simulink model "pdmRecipPump"  (R2021b)
settings: Solver=VariableStepAuto  StartTime=0.0  StopTime=2  RelTol=1e-3  EnableMultiTasking=on
undefined symbols (not defined in the file or in its folder): bearing_fault_frict_WKSP, bearing_visc_frict_WKSP, block_in_factor_WKSP, chkv_in_maxA_WKSP, noise_seed_offset_WKSP, smiData, TRP_Par, X, Y, Z
libraries: sm_lib x71, fl_lib x30, nesl_utility x13, sh_lib x8, simulink x7, ee_lib x2, Mech_Hydro_Elec_Multibody_Lib x2, sm_pump_triplex_lib x2
(part 2 of 4)

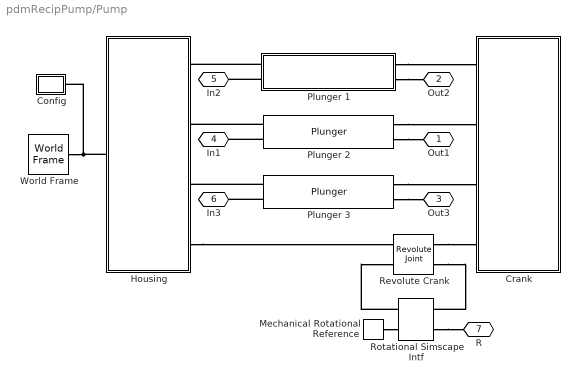
== system pdmRecipPump/Pump ==
  Config : Subsystem
  Crank : Subsystem  mask(Crankshaft){shaft_len=shaft_len_P, shaft_rad=shaft_rad_P, web_rad=web_rad_P, web_len=web_len_P, motor_shaft_rad=motor_shaft_rad_P, motor_shaft_len=motor_shaft_len_P, shaft_pos=shaft_pos_P, crank_rho=crank_rho_P, motor_shaft_clr=motor_shaft_clr_P, crank_clr=crank_clr_P, crank_opc=crank_opc_P}
      mask prompts: shaft_pos "Crankpin Axis Offset (m)"; crank_rho "Density (kg/m^3)"; motor_shaft_clr "Motor Shaft Color [RGB]"; crank_clr "Crank Color [RGB]"; crank_opc "Opacity (0-1)"
      mask help: Models pump crankshaft with three crankpins, each offset by 120 degrees from the crankshaft axis.
      mask DialogControl text_radius Prompt: Radius (m)
      mask DialogControl text_length Prompt: Length (m)
      mask DialogControl text_crankpin Prompt: Crankpin
      mask DialogControl text_web Prompt: Web
      mask DialogControl text_motor_shaft Prompt: Motor Shaft
      mask DialogControl cont_crank_vis Prompt: Crankshaft Visualization
      mask Display: image('sm_pump_triplex_Crank_IMAGE.png');
  Housing : Subsystem
      mask Display: image('sm_pump_triplex_Housing_IMAGE.png');
  Mechanical Rotational Reference : fl_lib/Mechanical/Rotational Elements/Mechanical Rotational Reference
  Plunger 1 : Subsystem  mask(Hydraulic Plunger){cyl_gap=cyl_gap_P, cyl_rad_out=cyl_rad_out_P, cyl_len=cyl_len_P, cyl_stroke=cyl_stroke_P, cyl_rad_in=0, cyl_xc_rev=0, cyl_frict_brkway_frc=cyl_frict_brkway_frc_P, cyl_frict_brkway_vel=cyl_frict_brkway_vel_P, cyl_frict_col_frc=cyl_frict_col_frc_P, cyl_frict_visc_coef=cyl_frict_visc_coef_P, cyl_rho=cyl_rho_P, cyl_clr=cyl_clr_P, cyl_opc=cyl_opc_P, cyl_xc=0, plgB_len=plgB_len_P, plgB_rad=plgB_rad_P, stem_len=stem_len_P, stem_rad=stem_rad_P, pin_len=pin_len_P, pin_rad=pin_rad_P, cup_rad_out=cup_rad_out_P, cup_thk=cup_thk_P, cup_len=cup_len_P, cup_pinOffset=cup_pinOffset_P, cup_rad_in=0, plg_rho=plg_rho_P, plg_clr=plg_clr_P, plg_opc=plg_opc_P, conrod_len=conrod_len_P, conrod_web_widP=conrod_web_widP_P, conrod_web_widC=conrod_web_widC_P, conrod_web_offC=0, conrod_web_offP=0, conrod_web_len=0, conrod_web_xc=0, conrod_ringC_wid=conrod_ringC_wid_P, conrod_ringP_wid=conrod_ringP_wid_P, crank_shaft_rad=crank_shaft_rad_P, conrod_ringC_or=0, conrod_ringP_or=0, conrod_ringC_xc_rev=0, conrod_ringP_xc_rev=0, conrod_thk=conrod_thk_P, conrod_rho=conrod_rho_P, conrod_clr=conrod_clr_P, conrod_opc=conrod_opc_P, chkv_in_maxA=chkv_in_maxA_P, chkv_out_maxA=chkv_out_maxA_P, chkv_in_crkP=chkv_in_crkP_P, chkv_out_crkP=chkv_out_crkP_P, chkv_in_maxOpenP=chkv_in_maxOpenP_P, chkv_out_maxOpenP=chkv_out_maxOpenP_P, chkv_vis_popup=Off, chkv_vis_rad_in=chkv_vis_rad_in_P, chkv_vis_rad_out=chkv_vis_rad_out_P, chkv_vis_clr_in=chkv_vis_clr_in_P, chkv_vis_clr_out=chkv_vis_clr_out_P, leak_cyl_popup=On, Run Time, leak_cyl_area=leak_cyl1_area, block_in_popup=On, Run Time, block_in_factor=block_in_cyl1_factor, seal_leak_vis_len=seal_leak_vis_len_P, seal_leak_vis_rad=seal_leak_vis_rad_P, seal_leak_vis_clr=seal_leak_vis_clr_P, seal_leak_vis_opc=0, inlet_obstr_len=inlet_obstr_len_P, inlet_obstr_rad=inlet_obstr_rad_P, inlet_obstr_xc_rev=0, inlet_obstr_clr=inlet_obstr_clr_P, inlet_obstr_opc=1}
      mask prompts: cyl_gap "Gap (m)"; cyl_rad_out "Outer radius (m)"; cyl_len "Length (m)"; cyl_stroke "Stroke (m)"; cyl_rad_in "Inner radius (m)"; cyl_xc_rev "Revolution Cross Section (m)"; cyl_frict_brkway_frc "Breakaway Friction Force (N)"; cyl_frict_brkway_vel "Breakaway Friction Velocity (m/s)"; cyl_frict_col_frc "Coulomb Friction Force (N)"; cyl_frict_visc_coef "Viscous Friction Coeff (N/(m/s))"; cyl_rho "Density (kg/m^3)"; cyl_clr "Color [RGB]"; cyl_opc "Opacity (0-1)"; cyl_xc "Cylinder Cross Section (m)"; cup_rad_out "Outer Radius (m)"; cup_thk "Wall Thickness (m)"; cup_len "Length(m)"; cup_pinOffset "Pin Offset (m)"; cup_rad_in "Inner Radius (m)"; plg_rho "Density (kg/m^3)"; plg_clr "Color [RGB]"; plg_opc "Opacity (0-1)"; conrod_len "Length, center-center (m)"; conrod_web_widP "Width, pin end (m)"; conrod_web_widC "Width, crank end (m)"; conrod_web_offC "Offset to shaft center (m)"; conrod_web_offP "Offset to pin center (m)"; conrod_web_len "Length web (m)"; conrod_web_xc "Extrusion cross section (m)"; conrod_ringC_wid "Crank Ring Width (m)"; conrod_ringP_wid "Pin Ring Width (m)"; crank_shaft_rad "Crank Shaft Radius (m)"; conrod_ringC_or "Outer Radius, Crank Ring"; conrod_ringP_or "Inner Radius, Pin Ring"; conrod_ringC_xc_rev "Crank Ring Cross Section (m)"; conrod_ringP_xc_rev "Pin Ring Cross Section (m)"; conrod_thk "Thickness (m)"; conrod_rho "Density (kg/m^3)"; conrod_clr "Color [RGB]"; conrod_opc "Opacity (0-1)"; chkv_vis_popup "Valve Visualization"; leak_cyl_popup "Seal Leak"; leak_cyl_area "Leak Area (m^2)"; block_in_popup "Blocked Inlet"; block_in_factor "Area Factor (0-1)"; seal_leak_vis_len "Length (m)"; seal_leak_vis_rad "Radius (m)"; seal_leak_vis_clr "Color [RGB]"; seal_leak_vis_opc "Opacity (0-1)"; inlet_obstr_len "Length (m)"; inlet_obstr_rad "Radius (m)"; inlet_obstr_xc_rev "Cross Section (m)"; inlet_obstr_clr "Color [RGB]"; inlet_obstr_opc "Opacity (0-1)"
      mask help: Models a single hydraulic plunger with hydraulic chamber. Two check valves control flow into and out of the hydraulic chamber. Degraded behavior can be modeled by enabling seal leakage and blocked inlet on the Faults tab. When "On, Run Time" is selected, MATLAB workspace variables set the parameters so that they can be tuned using Fast Restart.
      mask init:
      | % -- Configure submodels
      | % Fault: Seal Leak
      | if(leak_cyl_popup==1)
      |     set_param([gcb '/Seal Leak'],'OverrideUsingVariant','Off');
      |     seal_leak_vis_opc = 0;
      | elseif(leak_cyl_popup==2)
      |     set_param([gcb '/Seal Leak'],'OverrideUsingVariant','On');
      |     seal_leak_vis_opc = 1;
      | elseif(leak_cyl_popup==3)
      |     set_param([gcb '/Seal Leak'],'OverrideUsingVariant','Tune');
      |     seal_leak_vis_opc = 1;
      | end
      | 
      | % Fault: Blocked Inlet
      | inlet_obstr_xc_rev = [...
      |     inlet_obstr_rad                  -inlet_obstr_len/2;
      |     inlet_obstr_rad                   inlet_obstr_len/2;
      |     inlet_obstr_rad*block_in_factor   inlet_obstr_len/2;
      |     inlet_obstr_rad*block_in_factor  -inlet_obstr_len/2];
      | if(block_in_popup==1)
      |     set_param([gcb '/Check Valve Inlet'],...
      |         'area_max','chkv_in_maxA',...
      |         'area_max_conf','compiletime',...
      |         'BackgroundColor','[1 1 1]');
      |     inlet_obstr_opc = 0;
      | elseif(block_in_popup==2)
      |     set_param([gcb '/Check Valve Inlet'],...
      |         'area_max','chkv_in_maxA*block_in_factor',...
      |         'area_max_conf','compiletime',...
      |         'BackgroundColor','[1 0.9 0.9]');
      |     inlet_obstr_opc = 1;
      | elseif(block_in_popup==3)
      |     set_param([gcb '/Check Valve Inlet'],...
      |         'area_max','chkv_in_maxA_WKSP*block_in_factor_WKSP',...
      |         'area_max_conf','runtime',...
      |         'BackgroundColor','[1 0.9 0.9]');
      |     inlet_obstr_opc = 1;
      | end
      | 
      | % Turn on/off visualization
      | if(chkv_vis_popup==1)
      |     set_param([gcb '/Valve Visual'],'OverrideUsingVariant','Off');
      | elseif(chkv_vis_popup==2)
      |     set_param([gcb '/Valve Visual'],'OverrideUsingVariant','On');
      | end    
      | 
      | % -- Calculate derived parameters
      | % Cylinder: derived dimensions
      | cyl_rad_in  = plgB_rad + cyl_gap;
      | %cyl_len     = crank_shaft_pos*2+plgB_len;
      | 
      | % Cylinder: cross-section for rev
      | cyl_xc_rev = [...
      |     cyl_rad_out  -cyl_len/2
      |     cyl_rad_out   cyl_len/2
      |     cyl_rad_in    cyl_len/2
      |     cyl_rad_in   -cyl_len/2];
      | 
      | % Stem Cup: cross-section for rev
      | cup_rad_in = cup_rad_out-cup_thk;
      | cup_xc_rev = [...
      |     cup_rad_out  -cup_len/2
      |     cup_rad_out   cup_len/2
      |     cup_rad_in    cup_len/2
      |     cup_rad_in   -cup_len/2];
      | 
      | % Connecting Rod, Crank Ring: cross-section for rev
      | conrod_ringC_or = crank_shaft_rad + conrod_ringC_wid;
      | conrod_ringC_xc_rev = [...
      |     conrod_ringC_or -conrod_thk/2*1.005;
      |     conrod_ringC_or  conrod_thk/2*1.005;
      |     crank_shaft_rad  conrod_thk/2*1.005;
      |     crank_shaft_rad -conrod_thk/2*1.005];
      | 
      | % Connecting Rod, Pin ring: cross-section for rev
      | conrod_ringP_or = pin_rad + conrod_ringP_wid;
      | conrod_ringP_xc_rev = [...
      |     conrod_ringP_or -conrod_thk/2*1.005;
      |     conrod_ringP_or  conrod_thk/2*1.005;
      |     pin_rad          conrod_thk/2*1.005;
      |     pin_rad         -conrod_thk/2*1.005];
      | 
      | % Connecting Rod, Web: cross-section for extrusion
      | conrod_web_offC = crank_shaft_rad + conrod_ringC_wid/2;
      | conrod_web_offP = pin_rad         + conrod_ringP_wid/2;
      | conrod_web_len  = conrod_len - conrod_web_offP - conrod_web_offC;
      | conrod_web_xc = [...
      |     -conrod_web_len -conrod_web_widC;
      |      conrod_web_len -conrod_web_widP;
      |      conrod_web_len  conrod_web_widP;
      |     -conrod_web_len  conrod_web_widC]/2;
      mask TypeOptions chkv_vis_popup: Off | On
      mask TypeOptions leak_cyl_popup: Off | On | On, Run Time
      mask Callback leak_cyl_popup:
      | maskObj = Simulink.Mask.get(gcb);
      | leak_area_h = maskObj.getParameter('leak_cyl_area');
      | leak_text_h = maskObj.getDialogControl('leak_cyl_tune_text');
      | if (strcmp(get_param(gcb,'leak_cyl_popup'),'Off'))
      |     leak_area_h.Visible = 'off';
      |     leak_text_h.Visible = 'off';
      | elseif (strcmp(get_param(gcb,'leak_cyl_popup'),'On'))
      |     leak_area_h.Visible = 'on';
      |     leak_text_h.Visible = 'off';
      | elseif (strcmp(get_param(gcb,'leak_cyl_popup'),'On, Run Time'))
      |     leak_area_h.Visible = 'off';
      |     leak_text_h.Visible = 'on';
      | end
      | %clear maskObj leak_area_h leak_text_h
      mask TypeOptions block_in_popup: Off | On | On, Run Time
      mask Callback block_in_popup:
      | maskObj = Simulink.Mask.get(gcb);
      | block_fctr_h = maskObj.getParameter('block_in_factor');
      | block_text_h = maskObj.getDialogControl('block_in_tune_text');
      | if (strcmp(get_param(gcb,'block_in_popup'),'Off'))
      |     block_fctr_h.Visible = 'off';
      |     block_text_h.Visible = 'off';
      | elseif (strcmp(get_param(gcb,'block_in_popup'),'On'))
      |     block_fctr_h.Visible = 'on';
      |     block_text_h.Visible = 'off';
      | elseif (strcmp(get_param(gcb,'block_in_popup'),'On, Run Time'))
      |     block_fctr_h.Visible = 'off';
      |     block_text_h.Visible = 'on';
      | end
      | clear maskObj block_fctr_h block_text_h
      mask DialogControl tab_cylinder Prompt: Cylinder
      mask DialogControl cont_dims Prompt: Dimensions
      mask DialogControl cont_friction Prompt: Friction
      mask DialogControl tab_plunger Prompt: Plunger
      mask DialogControl text_length Prompt: Length (m)
      mask DialogControl text_radius Prompt: Radius (m)
      mask DialogControl text_base Prompt: Base
      mask DialogControl text_stem Prompt: Stem
      mask DialogControl text_pin Prompt: Pin
      mask DialogControl cont_cup Prompt: Cup
      mask DialogControl cont_plg_vis Prompt: Plunger Visualization
      mask DialogControl tab_conrod Prompt: Rod
      mask DialogControl cont_conrodWeb Prompt: Web
      mask DialogControl cont_conrodRings Prompt: Rings
      mask DialogControl cont_conrod_vis Prompt: Rod Visualization
      mask DialogControl tab_valves Prompt: Valves
      mask DialogControl text_open_inlet Prompt: Inlet
      mask DialogControl text_open_outlet Prompt: Outlet
      mask DialogControl text_open_maxA Prompt: Max Area (m)
      mask DialogControl text_open_crkP Prompt: Crack. Pr (Pa)
      mask DialogControl text_open_maxOpenP Prompt: Max Open. Pr. (Pa)
      mask DialogControl cont_valve_vis Prompt: Visualization Settings
      mask DialogControl text_valvis_inlet Prompt: Inlet
      mask DialogControl text_valvis_out Prompt: Outlet
      mask DialogControl text_valvis_rad Prompt: Radius (m)
      mask DialogControl text_valvis_clr Prompt: Color [RGB]
      mask DialogControl tab_faults Prompt: Faults
      mask DialogControl leak_cyl_tune_text Prompt: Set >> leak_cyl_area_WKSP
      mask DialogControl block_in_tune_text Prompt: Set >> block_in_factor_WKSP, chkv_out_maxA_WKSP
      mask DialogControl cont_seal_leak_vis Prompt: Seal Leak Visualization
      mask DialogControl cont_blocked_line_vis Prompt: Blocked Line Visualization
      mask Display: image('sm_pump_triplex_Plunger_IMAGE.png');
  Plunger 2 : sm_pump_triplex_lib/Plunger  cyl_gap=cyl_gap_P  cyl_rad_out=cyl_rad_out_P  cyl_len=cyl_len_P  cyl_stroke=cyl_stroke_P  cyl_rad_in=0  cyl_xc_rev=0  cyl_frict_brkway_frc=cyl_frict_brkway_frc_P  cyl_frict_brkway_vel=cyl_frict_brkway_vel_P  cyl_frict_col_frc=cyl_frict_col_frc_P  cyl_frict_visc_coef=cyl_frict_visc_coef_P  cyl_rho=cyl_rho_P  cyl_clr=cyl_clr_P  cyl_opc=cyl_opc_P  cyl_xc=0  plgB_len=plgB_len_P  plgB_rad=plgB_rad_P  stem_len=stem_len_P  stem_rad=stem_rad_P  pin_len=pin_len_P  pin_rad=pin_rad_P  cup_rad_out=cup_rad_out_P  cup_thk=cup_thk_P  cup_len=cup_len_P  cup_pinOffset=cup_pinOffset_P  cup_rad_in=0  plg_rho=plg_rho_P  plg_clr=plg_clr_P  plg_opc=plg_opc_P  conrod_len=conrod_len_P  conrod_web_widP=conrod_web_widP_P  conrod_web_widC=conrod_web_widC_P  conrod_web_offC=0  conrod_web_offP=0  conrod_web_len=0  conrod_web_xc=0  conrod_ringC_wid=conrod_ringC_wid_P  conrod_ringP_wid=conrod_ringP_wid_P  crank_shaft_rad=crank_shaft_rad_P  conrod_ringC_or=0  conrod_ringP_or=0  conrod_ringC_xc_rev=0  conrod_ringP_xc_rev=0  conrod_thk=conrod_thk_P  conrod_rho=conrod_rho_P  conrod_clr=conrod_clr_P  conrod_opc=conrod_opc_P  chkv_in_maxA=chkv_in_maxA_P  chkv_out_maxA=chkv_out_maxA_P  chkv_in_crkP=chkv_in_crkP_P  chkv_out_crkP=chkv_out_crkP_P  chkv_in_maxOpenP=chkv_in_maxOpenP_P  chkv_out_maxOpenP=chkv_out_maxOpenP_P  chkv_vis_popup=Off  chkv_vis_rad_in=chkv_vis_rad_in_P  chkv_vis_rad_out=chkv_vis_rad_out_P  chkv_vis_clr_in=chkv_vis_clr_in_P  chkv_vis_clr_out=chkv_vis_clr_out_P  leak_cyl_popup=Off  leak_cyl_area=leak_cyl2_area  block_in_popup=Off  block_in_factor=block_in_cyl2_factor  seal_leak_vis_len=seal_leak_vis_len_P  seal_leak_vis_rad=seal_leak_vis_rad_P  seal_leak_vis_clr=seal_leak_vis_clr_P  seal_leak_vis_opc=0  inlet_obstr_len=inlet_obstr_len_P  inlet_obstr_rad=inlet_obstr_rad_P  inlet_obstr_xc_rev=0  inlet_obstr_clr=inlet_obstr_clr_P  inlet_obstr_opc=1
  Plunger 3 : sm_pump_triplex_lib/Plunger  cyl_gap=cyl_gap_P  cyl_rad_out=cyl_rad_out_P  cyl_len=cyl_len_P  cyl_stroke=cyl_stroke_P  cyl_rad_in=0  cyl_xc_rev=0  cyl_frict_brkway_frc=cyl_frict_brkway_frc_P  cyl_frict_brkway_vel=cyl_frict_brkway_vel_P  cyl_frict_col_frc=cyl_frict_col_frc_P  cyl_frict_visc_coef=cyl_frict_visc_coef_P  cyl_rho=cyl_rho_P  cyl_clr=cyl_clr_P  cyl_opc=cyl_opc_P  cyl_xc=0  plgB_len=plgB_len_P  plgB_rad=plgB_rad_P  stem_len=stem_len_P  stem_rad=stem_rad_P  pin_len=pin_len_P  pin_rad=pin_rad_P  cup_rad_out=cup_rad_out_P  cup_thk=cup_thk_P  cup_len=cup_len_P  cup_pinOffset=cup_pinOffset_P  cup_rad_in=0  plg_rho=plg_rho_P  plg_clr=plg_clr_P  plg_opc=plg_opc_P  conrod_len=conrod_len_P  conrod_web_widP=conrod_web_widP_P  conrod_web_widC=conrod_web_widC_P  conrod_web_offC=0  conrod_web_offP=0  conrod_web_len=0  conrod_web_xc=0  conrod_ringC_wid=conrod_ringC_wid_P  conrod_ringP_wid=conrod_ringP_wid_P  crank_shaft_rad=crank_shaft_rad_P  conrod_ringC_or=0  conrod_ringP_or=0  conrod_ringC_xc_rev=0  conrod_ringP_xc_rev=0  conrod_thk=conrod_thk_P  conrod_rho=conrod_rho_P  conrod_clr=conrod_clr_P  conrod_opc=conrod_opc_P  chkv_in_maxA=chkv_in_maxA_P  chkv_out_maxA=chkv_out_maxA_P  chkv_in_crkP=chkv_in_crkP_P  chkv_out_crkP=chkv_out_crkP_P  chkv_in_maxOpenP=chkv_in_maxOpenP_P  chkv_out_maxOpenP=chkv_out_maxOpenP_P  chkv_vis_popup=Off  chkv_vis_rad_in=chkv_vis_rad_in_P  chkv_vis_rad_out=chkv_vis_rad_out_P  chkv_vis_clr_in=chkv_vis_clr_in_P  chkv_vis_clr_out=chkv_vis_clr_out_P  leak_cyl_popup=Off  leak_cyl_area=leak_cyl3_area  block_in_popup=Off  block_in_factor=block_in_cyl3_factor  seal_leak_vis_len=seal_leak_vis_len_P  seal_leak_vis_rad=seal_leak_vis_rad_P  seal_leak_vis_clr=seal_leak_vis_clr_P  seal_leak_vis_opc=0  inlet_obstr_len=inlet_obstr_len_P  inlet_obstr_rad=inlet_obstr_rad_P  inlet_obstr_xc_rev=0  inlet_obstr_clr=inlet_obstr_clr_P  inlet_obstr_opc=1
  Revolute Crank : sm_lib/Joints/Revolute Joint  JointMode=Normal  SenseConstraintForce=off  SenseConstraintForceX=off  SenseConstraintForceY=off  SenseConstraintForceZ=off  SenseConstraintTorque=off  SenseConstraintTorqueX=off  SenseConstraintTorqueY=off  SenseConstraintTorqueZ=off  SenseTotalForce=off  SenseTotalForceX=off  SenseTotalForceY=off  SenseTotalForceZ=off  SenseTotalTorque=off  SenseTotalTorqueX=off  SenseTotalTorqueY=off  SenseTotalTorqueZ=off  CompositeWrenchDir=FollowerOnBase  CompositeWrenchFrame=BaseFrame  EquilibriumPosition=0  EquilibriumPositionUnits=deg  SpringStiffness=0  SpringStiffnessUnits=N*m/deg  DampingCoefficient=bearing_visc_frict_WKSP+bearing_fault_frict_WKSP  DampingCoefficientUnits=N*m/(deg/s)  TorqueActuationMode=InputTorque  MotionActuationMode=ComputedMotion  SensePosition=off  SenseVelocity=on  SenseAcceleration=off  SenseTorqueForce=off  SenseLowerLimitTorqueForce=off  SenseUpperLimitTorqueForce=off  LowerLimitSpecify=off  LowerLimitBound=-90  LowerLimitBoundUnits=deg  LowerLimitStiffness=1e4  LowerLimitStiffnessUnits=N*m/deg  LowerLimitDamping=10  LowerLimitDampingUnits=N*m/(deg/s)  LowerLimitTransitionRegionWidth=0.1  LowerLimitTransitionRegionWidthUnits=deg  UpperLimitSpecify=off  UpperLimitBound=90  UpperLimitBoundUnits=deg  UpperLimitStiffness=1e4  UpperLimitStiffnessUnits=N*m/deg  UpperLimitDamping=10  UpperLimitDampingUnits=N*m/(deg/s)  UpperLimitTransitionRegionWidth=0.1  UpperLimitTransitionRegionWidthUnits=deg  PositionTargetSpecify=off  PositionTargetPriority=High  PositionTargetValue=0  PositionTargetValueUnits=deg  VelocityTargetSpecify=off  VelocityTargetPriority=High  VelocityTargetValue=0  VelocityTargetValueUnits=deg/s
  Rotational Simscape Intf : Mech_Hydro_Elec_Multibody_Lib/Interfaces/Rotational Simscape Intf  SystemSampleTime=-1  VariantActivationTime=update diagram  Latency=0  AutoFrameSizeCalculation=off
  World Frame : sm_lib/Frames and Transforms/World Frame
  Out1 : PMIOPort  Side=Right
  Out2 : PMIOPort  Port=2  Side=Right
  Out3 : PMIOPort  Port=3  Side=Right
  In1 : PMIOPort  Port=4  Side=Right
  In2 : PMIOPort  Port=5  Side=Right
  In3 : PMIOPort  Port=6  Side=Right
  R : PMIOPort  Port=7  Side=Left
  connections:
  Housing/LConn1 -- World Frame/RConn1 -- Config/RConn1
  Plunger 2/LConn1 -- Housing/RConn2
  Plunger 1/LConn2 -- In2/RConn1
  Plunger 1/RConn1 -- Crank/LConn1
  Plunger 2/RConn1 -- Crank/LConn2
  Plunger 3/LConn2 -- In3/RConn1
  Plunger 3/RConn2 -- Out3/RConn1
  Revolute Crank/RConn2 -- Rotational Simscape Intf/RConn1
  Plunger 1/LConn1 -- Housing/RConn1
  Plunger 2/LConn2 -- In1/RConn1
  Plunger 3/LConn1 -- Housing/RConn3
  Mechanical Rotational Reference/LConn1 -- Rotational Simscape Intf/LConn2
  Rotational Simscape Intf/LConn1 -- Revolute Crank/LConn2
  Housing/RConn4 -- Revolute Crank/LConn1
  Revolute Crank/RConn1 -- Crank/LConn4
  Plunger 1/RConn2 -- Out2/RConn1
  Plunger 2/RConn2 -- Out1/RConn1
  Plunger 3/RConn1 -- Crank/LConn3
  Rotational Simscape Intf/RConn2 -- R/RConn1

== system pdmRecipPump/Sensing Current ==
  Current Sensor : fl_lib/Electrical/Electrical Sensors/Current Sensor
  Current with Noise : Scope  NumInputPorts=2
  Measurement Noise : simulink/Sources/Band-Limited White Noise  Cov=TRP_Par.Sensors.i.Np  Ts=TRP_Par.Sensors.i.Ts  seed=TRP_Par.Sensors.i.Seed+noise_seed_offset_WKSP
  PS-Simulink Converter : nesl_utility/PS-Simulink Converter  PhysicalDomain=network_engine_domain  SubClassName=ps_output  LeftPortType=input  RightPortType=output  PseudoPeriodic=off  Frequencies=[]  Unit=1  AffineConversion=off
      settings: SourceProductBaseCode=PW,SS
  Sum1 : Sum  Inputs=++|
  Zero-Order Hold : ZeroOrderHold  SampleTime=TRP_Par.Sensors.i.Ts
  - : PMIOPort  Side=Right
  + : PMIOPort  Port=2  Side=Left
  wires:
  Measurement Noise/1 -> Sum1/1  "Noise"
  Sum1/1 -> Zero-Order Hold/1
  PS-Simulink Converter/1 -> Sum1/2, Current with Noise/2
  Zero-Order Hold/1 -> Current with Noise/1
  connections:
  PS-Simulink Converter/LConn1 -- Current Sensor/RConn1
  +/RConn1 -- Current Sensor/LConn1
  Current Sensor/RConn2 -- -/RConn1

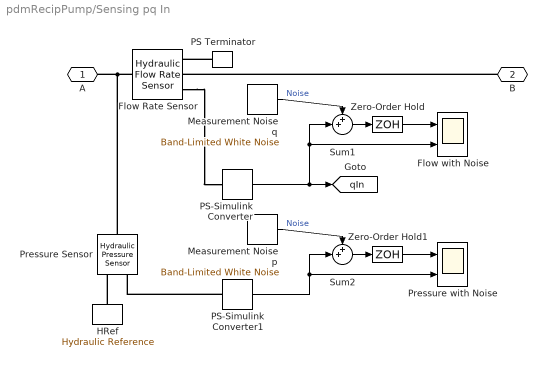
== system pdmRecipPump/Sensing pq In ==
  Flow Rate Sensor : fl_lib/Hydraulic/Hydraulic Sensors/Hydraulic Flow Rate Sensor
  Flow with Noise : Scope  NumInputPorts=2
  HRef : fl_lib/Hydraulic/Hydraulic Elements/Hydraulic Reference
  Measurement Noise p : simulink/Sources/Band-Limited White Noise  Cov=TRP_Par.Sensors.p.Np  Ts=TRP_Par.Sensors.p.Ts  seed=TRP_Par.Sensors.p.Seed+noise_seed_offset_WKSP
  Measurement Noise q : simulink/Sources/Band-Limited White Noise  Cov=TRP_Par.Sensors.q.Np  Ts=TRP_Par.Sensors.q.Ts  seed=TRP_Par.Sensors.q.Seed+noise_seed_offset_WKSP
  PS Terminator : fl_lib/Physical Signals/Sinks/PS Terminator
  PS-Simulink Converter : nesl_utility/PS-Simulink Converter  PhysicalDomain=network_engine_domain  SubClassName=ps_output  LeftPortType=input  RightPortType=output  PseudoPeriodic=off  Frequencies=[]  Unit=lpm  AffineConversion=off
      settings: SourceProductBaseCode=PW,SS
  PS-Simulink Converter1 : nesl_utility/PS-Simulink Converter  PhysicalDomain=network_engine_domain  SubClassName=ps_output  LeftPortType=input  RightPortType=output  PseudoPeriodic=off  Frequencies=[]  Unit=bar  AffineConversion=off
      settings: SourceProductBaseCode=PW,SS
  Pressure Sensor : fl_lib/Hydraulic/Hydraulic Sensors/Hydraulic Pressure Sensor
  Pressure with Noise : Scope  NumInputPorts=2
  Sum1 : Sum  Inputs=++|
  Sum2 : Sum  Inputs=++|
  Zero-Order Hold : ZeroOrderHold  SampleTime=TRP_Par.Sensors.q.Ts
  Zero-Order Hold1 : ZeroOrderHold  SampleTime=TRP_Par.Sensors.p.Ts
  A : PMIOPort  Side=Left
  B : PMIOPort  Port=2  Side=Right
  tag scope: qIn=global
  wires:
  Zero-Order Hold1/1 -> Pressure with Noise/1
  Measurement Noise p/1 -> Sum2/1  "Noise"
  PS-Simulink Converter1/1 -> Pressure with Noise/2, Sum2/2
  Sum2/1 -> Zero-Order Hold1/1
  Zero-Order Hold/1 -> Flow with Noise/1
  Sum1/1 -> Zero-Order Hold/1
  Measurement Noise q/1 -> Sum1/1  "Noise"
  PS-Simulink Converter/1 -> [qIn], Flow with Noise/2, Sum1/2
  connections:
  PS-Simulink Converter1/LConn1 -- Pressure Sensor/RConn2
  HRef/LConn1 -- Pressure Sensor/RConn1
  Flow Rate Sensor/RConn1 -- PS-Simulink Converter/LConn1
  B/RConn1 -- Flow Rate Sensor/RConn2
  Pressure Sensor/LConn1 -- Flow Rate Sensor/LConn1 -- A/RConn1
  PS Terminator/LConn1 -- Flow Rate Sensor/RConn3

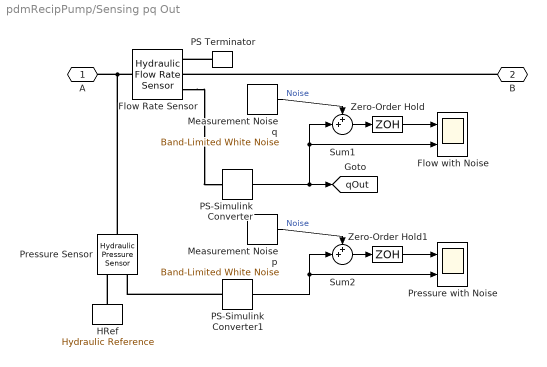
== system pdmRecipPump/Sensing pq Out ==
  Flow Rate Sensor : fl_lib/Hydraulic/Hydraulic Sensors/Hydraulic Flow Rate Sensor
  Flow with Noise : Scope  NumInputPorts=2
  HRef : fl_lib/Hydraulic/Hydraulic Elements/Hydraulic Reference
  Measurement Noise p : simulink/Sources/Band-Limited White Noise  Cov=TRP_Par.Sensors.p.Np  Ts=TRP_Par.Sensors.p.Ts  seed=TRP_Par.Sensors.p.Seed+noise_seed_offset_WKSP
  Measurement Noise q : simulink/Sources/Band-Limited White Noise  Cov=TRP_Par.Sensors.q.Np  Ts=TRP_Par.Sensors.q.Ts  seed=TRP_Par.Sensors.q.Seed+noise_seed_offset_WKSP
  PS Terminator : fl_lib/Physical Signals/Sinks/PS Terminator
  PS-Simulink Converter : nesl_utility/PS-Simulink Converter  PhysicalDomain=network_engine_domain  SubClassName=ps_output  LeftPortType=input  RightPortType=output  PseudoPeriodic=off  Frequencies=[]  Unit=lpm  AffineConversion=off
      settings: SourceProductBaseCode=PW,SS
  PS-Simulink Converter1 : nesl_utility/PS-Simulink Converter  PhysicalDomain=network_engine_domain  SubClassName=ps_output  LeftPortType=input  RightPortType=output  PseudoPeriodic=off  Frequencies=[]  Unit=bar  AffineConversion=off
      settings: SourceProductBaseCode=PW,SS
  Pressure Sensor : fl_lib/Hydraulic/Hydraulic Sensors/Hydraulic Pressure Sensor
  Pressure with Noise : Scope  NumInputPorts=2
  Sum1 : Sum  Inputs=++|
  Sum2 : Sum  Inputs=++|
  Zero-Order Hold : ZeroOrderHold  SampleTime=TRP_Par.Sensors.q.Ts
  Zero-Order Hold1 : ZeroOrderHold  SampleTime=TRP_Par.Sensors.p.Ts
  A : PMIOPort  Side=Left
  B : PMIOPort  Port=2  Side=Right
  tag scope: qOut=global
  wires:
  PS-Simulink Converter/1 -> Sum1/2, Flow with Noise/2, [qOut]
  Measurement Noise q/1 -> Sum1/1  "Noise"
  Sum1/1 -> Zero-Order Hold/1
  Zero-Order Hold/1 -> Flow with Noise/1
  Sum2/1 -> Zero-Order Hold1/1
  PS-Simulink Converter1/1 -> Sum2/2, Pressure with Noise/2
  Measurement Noise p/1 -> Sum2/1  "Noise"
  Zero-Order Hold1/1 -> Pressure with Noise/1
  connections:
  PS Terminator/LConn1 -- Flow Rate Sensor/RConn3
  Flow Rate Sensor/LConn1 -- Pressure Sensor/LConn1 -- A/RConn1
  B/RConn1 -- Flow Rate Sensor/RConn2
  Flow Rate Sensor/RConn1 -- PS-Simulink Converter/LConn1
  HRef/LConn1 -- Pressure Sensor/RConn1
  PS-Simulink Converter1/LConn1 -- Pressure Sensor/RConn2

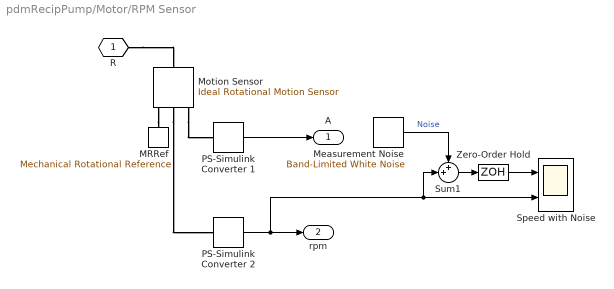
== system pdmRecipPump/Motor/RPM Sensor ==
  MRRef : fl_lib/Mechanical/Rotational Elements/Mechanical Rotational Reference
  Measurement Noise : simulink/Sources/Band-Limited White Noise  Cov=TRP_Par.Sensors.w.Np  Ts=TRP_Par.Sensors.w.Ts  seed=TRP_Par.Sensors.w.Seed+noise_seed_offset_WKSP
  Motion Sensor : fl_lib/Mechanical/Mechanical Sensors/Ideal Rotational Motion Sensor  wrap_angle=simscape.enum.onoff.off  offset=0 rad
  PS-Simulink Converter 1 : nesl_utility/PS-Simulink Converter  PhysicalDomain=network_engine_domain  SubClassName=ps_output  LeftPortType=input  RightPortType=output  PseudoPeriodic=off  Frequencies=[]  Unit=deg  AffineConversion=off
      settings: SourceProductBaseCode=PW,SS
  PS-Simulink Converter 2 : nesl_utility/PS-Simulink Converter  PhysicalDomain=network_engine_domain  SubClassName=ps_output  LeftPortType=input  RightPortType=output  PseudoPeriodic=off  Frequencies=[]  Unit=rpm  AffineConversion=off
      settings: SourceProductBaseCode=PW,SS
  Speed with Noise : Scope  NumInputPorts=2
  Sum1 : Sum  Inputs=++|
  Zero-Order Hold : ZeroOrderHold  SampleTime=TRP_Par.Sensors.w.Ts
  R : PMIOPort  Side=Left
  A : Outport  VectorParamsAs1DForOutWhenUnconnected=off
  rpm : Outport  Port=2  VectorParamsAs1DForOutWhenUnconnected=off
  wires:
  PS-Simulink Converter 1/1 -> A/1
  Sum1/1 -> Zero-Order Hold/1
  Zero-Order Hold/1 -> Speed with Noise/1
  PS-Simulink Converter 2/1 -> Sum1/2, Speed with Noise/2, rpm/1
  Measurement Noise/1 -> Sum1/1  "Noise"
  connections:
  Motion Sensor/RConn2 -- PS-Simulink Converter 2/LConn1
  Motion Sensor/RConn1 -- MRRef/LConn1
  R/RConn1 -- Motion Sensor/LConn1
  Motion Sensor/RConn3 -- PS-Simulink Converter 1/LConn1

== system pdmRecipPump/Motor/Speed Controller ==
  rpm_ref : Inport
  rpm : Inport  Port=2
  Integrator : Integrator  LimitOutput=on  UpperSaturationLimit=40  LowerSaturationLimit=-40
      settings: AttributesFormatString=Saturate: [%<LowerSaturationLimit>, %<UpperSaturationLimit>]
  Ki : Gain  Gain=0.002
  Kp : Gain  Gain=0.02*2
  Lowpass Filter : TransferFcn  Denominator=[1/(2*pi*200) 1]
  Sum : Sum  Inputs=-+|
  Sum1 : Sum  Inputs=++|
  Torque Limits : Saturate  UpperLimit=400  LowerLimit=-400
  T_ref : Outport  VectorParamsAs1DForOutWhenUnconnected=off
  wires:
  rpm_ref/1 -> Sum/2
  rpm/1 -> Lowpass Filter/1
  Sum1/1 -> Torque Limits/1
  Sum/1 -> Ki/1, Kp/1
  Ki/1 -> Integrator/1
  Kp/1 -> Sum1/2
  Integrator/1 -> Sum1/1
  Lowpass Filter/1 -> Sum/1
  Torque Limits/1 -> T_ref/1

== system pdmRecipPump/Motor/Windings ==
  T_ref : Inport
  deg : Inport  Port=2
  Constant : Constant  Value=winding_fault_enable
  Constant1 : Constant
  Enable if rotor angle 0-240 Deg : Subsystem
  Product : Product
  Switch : Switch  Criteria=u2 > Threshold  Threshold=1.5
  Unit Delay : UnitDelay  SampleTime=0.001  HasFrameUpgradeWarning=on
  Trq : Outport  VectorParamsAs1DForOutWhenUnconnected=off
  wires:
  Product/1 -> Trq/1
  T_ref/1 -> Product/1
  Constant/1 -> Switch/2
  Constant1/1 -> Switch/3
  Switch/1 -> Product/2
  deg/1 -> Unit Delay/1
  Enable if rotor angle 0-240 Deg/1(En) -> Switch/1
  Unit Delay/1 -> Enable if rotor angle 0-240 Deg/1(Ang)

== system pdmRecipPump/Pump/Config ==
  Mechanism Configuration : sm_lib/Utilities/Mechanism Configuration  UniformGravity=Constant  GravityVector=[0 -1 0]*9.80665  GravityUnits=m/s^2  LinearizationDelta=0.001  JointModeTransitionNonlinearIterations=2
  Solver Configuration : nesl_utility/Solver Configuration  PhysicalDomain=network_engine_domain  SubClassName=solver  LeftPortType=input  RightPortType=generic  Tones=[]  Harmonics=[]  SimulateNoise=off  Profile=off  UseLocalSampling=off  EnableSwitchedLinearOptims=on  FrequencyDomain=off  UseCCode=off  RelTol=0.001  AbsTol=1e-06  MinStep=1e-09  ToWorkspace=off  RevertToSquareIcSolve=off  NumHomotopyIterations=100  PhasorMode=off  PhasorModeNumHarmonics=1  DoDC=off  ResidualTolerance=1e-10  UseLocalSolver=off  LocalSolverChoice=NE_BACKWARD_EULER_ADVANCER  LocalSolverSampleTime=0.001  DoFixedCost=off  MaxNonlinIter=3  MaxModeIter=2  ComputeImpulses=off  ImpulseIterations=2  LinearAlgebra=Sparse  EquationFormulation=NE_TIME_EF  DelaysMemoryBudget=1024  AutomaticFiltering=on  FilteringTimeConstant=0.001  PartitionStorageMethod=AS_NEEDED  PartitionMemoryBudget=1024  PartitionMethod=FAST
      settings: SourceProductBaseCode=PW,SS
  C : PMIOPort  Side=Right
  connections:
  Solver Configuration/RConn1 -- C/RConn1 -- Mechanism Configuration/RConn1

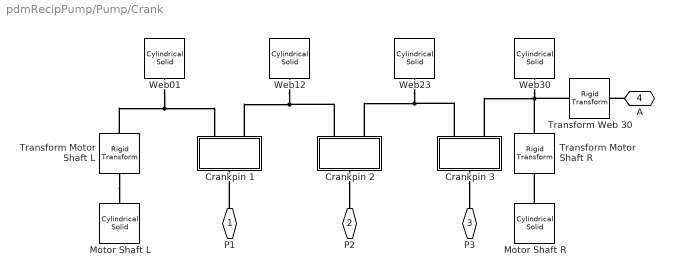
== system pdmRecipPump/Pump/Crank ==
  Crankpin 1 : Subsystem
  Crankpin 2 : Subsystem
  Crankpin 3 : Subsystem
  Motor Shaft L : sm_lib/Body Elements/Cylindrical Solid  GraphicAmbientColor=[0.15 0.15 0.15 1.0]  BasedOnType=Density  CenterOfMass=[0 0 0]  CenterOfMassUnits=m  GraphicDiffuseColor=motor_shaft_clr  CylinderLength=motor_shaft_len  CylinderLengthUnits=m  CylinderRadius=motor_shaft_rad  CylinderRadiusUnits=m  Density=crank_rho  DensityUnits=kg/m^3  DoExposeReferenceFrame=on  GraphicEmissiveColor=[0.0 0.0 0.0 1.0]  ExportEntireGeometry=off  SerializedFrames=<Frames/>  MarkerShape=Sphere  MarkerSize=10  GraphicType=FromGeometry  InertiaType=CalculateFromGeometry  Mass=1  MassUnits=kg  MomentsOfInertia=[1 1 1]  MomentsOfInertiaUnits=kg*m^2  GraphicOpacity=crank_opc  ProductsOfInertia=[1 1 1]  ProductsOfInertiaUnits=kg*m^2  GraphicShininess=75  GraphicSpecularColor=[0.5 0.5 0.5 1.0]  GraphicVisPropType=SimpleVisualProperties
  Motor Shaft R : sm_lib/Body Elements/Cylindrical Solid  GraphicAmbientColor=[0.15 0.15 0.15 1.0]  BasedOnType=Density  CenterOfMass=[0 0 0]  CenterOfMassUnits=m  GraphicDiffuseColor=motor_shaft_clr  CylinderLength=motor_shaft_len  CylinderLengthUnits=m  CylinderRadius=motor_shaft_rad  CylinderRadiusUnits=m  Density=crank_rho  DensityUnits=kg/m^3  DoExposeReferenceFrame=on  GraphicEmissiveColor=[0.0 0.0 0.0 1.0]  ExportEntireGeometry=off  SerializedFrames=<Frames/>  MarkerShape=Sphere  MarkerSize=10  GraphicType=FromGeometry  InertiaType=CalculateFromGeometry  Mass=1  MassUnits=kg  MomentsOfInertia=[1 1 1]  MomentsOfInertiaUnits=kg*m^2  GraphicOpacity=crank_opc  ProductsOfInertia=[1 1 1]  ProductsOfInertiaUnits=kg*m^2  GraphicShininess=75  GraphicSpecularColor=[0.5 0.5 0.5 1.0]  GraphicVisPropType=SimpleVisualProperties
  Transform Motor Shaft L : sm_lib/Frames and Transforms/Rigid Transform  TranslationMethod=StandardAxis  TranslationStandardOffset=motor_shaft_len/2  TranslationLengthUnit=m  TranslationStandardAxis=+Z  TranslationCartesianOffset=[0 0 0]  TranslationROffset=0  TranslationROffsetUnits=m  TranslationZOffset=0  TranslationZOffsetUnits=m  TranslationThetaOffset=0  TranslationThetaOffsetUnits=deg  RotationMethod=None  RotationAngleUnits=deg  RotationStandardAxis=+Z  RotationAngle=0.0  RotationArbitraryAxis=[0 0 1]  FollAlignAxisA=+X  BaseAlignAxisA=+Y  FollAlignAxisB=+Y  BaseAlignAxisB=+Z  RotationSequenceAxes=FollowerAxes  RotationSequence=XYX  RotationSequenceAngles=[0 0 0]  RotationSequenceAnglesUnits=deg  RotationMatrix=[1 0 0; 0 1 0; 0 0 1]
  Transform Motor Shaft R : sm_lib/Frames and Transforms/Rigid Transform  TranslationMethod=StandardAxis  TranslationStandardOffset=motor_shaft_len/2  TranslationLengthUnit=m  TranslationStandardAxis=+Z  TranslationCartesianOffset=[0 0 0]  TranslationROffset=0  TranslationROffsetUnits=m  TranslationZOffset=0  TranslationZOffsetUnits=m  TranslationThetaOffset=0  TranslationThetaOffsetUnits=deg  RotationMethod=None  RotationAngleUnits=deg  RotationStandardAxis=+Z  RotationAngle=0.0  RotationArbitraryAxis=[0 0 1]  FollAlignAxisA=+X  BaseAlignAxisA=+Y  FollAlignAxisB=+Y  BaseAlignAxisB=+Z  RotationSequenceAxes=FollowerAxes  RotationSequence=XYX  RotationSequenceAngles=[0 0 0]  RotationSequenceAnglesUnits=deg  RotationMatrix=[1 0 0; 0 1 0; 0 0 1]
  Transform Web 30 : sm_lib/Frames and Transforms/Rigid Transform  TranslationMethod=StandardAxis  TranslationStandardOffset=shaft_len*1.5  TranslationLengthUnit=m  TranslationStandardAxis=+Z  TranslationCartesianOffset=[0 0 0]  TranslationROffset=0  TranslationROffsetUnits=m  TranslationZOffset=0  TranslationZOffsetUnits=m  TranslationThetaOffset=0  TranslationThetaOffsetUnits=deg  RotationMethod=None  RotationAngleUnits=deg  RotationStandardAxis=+Z  RotationAngle=0.0  RotationArbitraryAxis=[0 0 1]  FollAlignAxisA=+X  BaseAlignAxisA=+Y  FollAlignAxisB=+Y  BaseAlignAxisB=+Z  RotationSequenceAxes=FollowerAxes  RotationSequence=XYX  RotationSequenceAngles=[0 0 0]  RotationSequenceAnglesUnits=deg  RotationMatrix=[1 0 0; 0 1 0; 0 0 1]
  Web01 : sm_lib/Body Elements/Cylindrical Solid  GraphicAmbientColor=[0.15 0.15 0.15 1.0]  BasedOnType=Density  CenterOfMass=[0 0 0]  CenterOfMassUnits=m  GraphicDiffuseColor=crank_clr  CylinderLength=web_len  CylinderLengthUnits=m  CylinderRadius=web_rad  CylinderRadiusUnits=m  Density=crank_rho  DensityUnits=kg/m^3  DoExposeReferenceFrame=on  GraphicEmissiveColor=[0.0 0.0 0.0 1.0]  ExportEntireGeometry=off  SerializedFrames=<Frames/>  MarkerShape=Sphere  MarkerSize=10  GraphicType=FromGeometry  InertiaType=CalculateFromGeometry  Mass=1  MassUnits=kg  MomentsOfInertia=[1 1 1]  MomentsOfInertiaUnits=kg*m^2  GraphicOpacity=crank_opc  ProductsOfInertia=[1 1 1]  ProductsOfInertiaUnits=kg*m^2  GraphicShininess=75  GraphicSpecularColor=[0.5 0.5 0.5 1.0]  GraphicVisPropType=SimpleVisualProperties
  Web12 : sm_lib/Body Elements/Cylindrical Solid  GraphicAmbientColor=[0.15 0.15 0.15 1.0]  BasedOnType=Density  CenterOfMass=[0 0 0]  CenterOfMassUnits=m  GraphicDiffuseColor=crank_clr  CylinderLength=web_len  CylinderLengthUnits=m  CylinderRadius=web_rad  CylinderRadiusUnits=m  Density=crank_rho  DensityUnits=kg/m^3  DoExposeReferenceFrame=on  GraphicEmissiveColor=[0.0 0.0 0.0 1.0]  ExportEntireGeometry=off  SerializedFrames=<Frames/>  MarkerShape=Sphere  MarkerSize=10  GraphicType=FromGeometry  InertiaType=CalculateFromGeometry  Mass=1  MassUnits=kg  MomentsOfInertia=[1 1 1]  MomentsOfInertiaUnits=kg*m^2  GraphicOpacity=crank_opc  ProductsOfInertia=[1 1 1]  ProductsOfInertiaUnits=kg*m^2  GraphicShininess=75  GraphicSpecularColor=[0.5 0.5 0.5 1.0]  GraphicVisPropType=SimpleVisualProperties
  Web23 : sm_lib/Body Elements/Cylindrical Solid  GraphicAmbientColor=[0.15 0.15 0.15 1.0]  BasedOnType=Density  CenterOfMass=[0 0 0]  CenterOfMassUnits=m  GraphicDiffuseColor=crank_clr  CylinderLength=web_len  CylinderLengthUnits=m  CylinderRadius=web_rad  CylinderRadiusUnits=m  Density=crank_rho  DensityUnits=kg/m^3  DoExposeReferenceFrame=on  GraphicEmissiveColor=[0.0 0.0 0.0 1.0]  ExportEntireGeometry=off  SerializedFrames=<Frames/>  MarkerShape=Sphere  MarkerSize=10  GraphicType=FromGeometry  InertiaType=CalculateFromGeometry  Mass=1  MassUnits=kg  MomentsOfInertia=[1 1 1]  MomentsOfInertiaUnits=kg*m^2  GraphicOpacity=crank_opc  ProductsOfInertia=[1 1 1]  ProductsOfInertiaUnits=kg*m^2  GraphicShininess=75  GraphicSpecularColor=[0.5 0.5 0.5 1.0]  GraphicVisPropType=SimpleVisualProperties
  Web30 : sm_lib/Body Elements/Cylindrical Solid  GraphicAmbientColor=[0.15 0.15 0.15 1.0]  BasedOnType=Density  CenterOfMass=[0 0 0]  CenterOfMassUnits=m  GraphicDiffuseColor=crank_clr  CylinderLength=web_len  CylinderLengthUnits=m  CylinderRadius=web_rad  CylinderRadiusUnits=m  Density=crank_rho  DensityUnits=kg/m^3  DoExposeReferenceFrame=on  GraphicEmissiveColor=[0.0 0.0 0.0 1.0]  ExportEntireGeometry=off  SerializedFrames=<Frames/>  MarkerShape=Sphere  MarkerSize=10  GraphicType=FromGeometry  InertiaType=CalculateFromGeometry  Mass=1  MassUnits=kg  MomentsOfInertia=[1 1 1]  MomentsOfInertiaUnits=kg*m^2  GraphicOpacity=crank_opc  ProductsOfInertia=[1 1 1]  ProductsOfInertiaUnits=kg*m^2  GraphicShininess=75  GraphicSpecularColor=[0.5 0.5 0.5 1.0]  GraphicVisPropType=SimpleVisualProperties
  P1 : PMIOPort  Side=Left
  P2 : PMIOPort  Port=2  Side=Left
  P3 : PMIOPort  Port=3  Side=Left
  A : PMIOPort  Port=4  Side=Left
  connections:
  Crankpin 2/LConn2 -- Web23/RConn1 -- Crankpin 3/LConn1
  Motor Shaft R/RConn1 -- Transform Motor Shaft R/RConn1
  Crankpin 1/LConn2 -- Web12/RConn1 -- Crankpin 2/LConn1
  Crankpin 2/RConn1 -- P2/RConn1
  Web01/RConn1 -- Transform Motor Shaft L/RConn1 -- Crankpin 1/LConn1
  P1/RConn1 -- Crankpin 1/RConn1
  Crankpin 3/RConn1 -- P3/RConn1
  Transform Motor Shaft R/LConn1 -- Transform Web 30/RConn1 -- Web30/RConn1 -- Crankpin 3/LConn2
  Transform Motor Shaft L/LConn1 -- Motor Shaft L/RConn1
  A/RConn1 -- Transform Web 30/LConn1

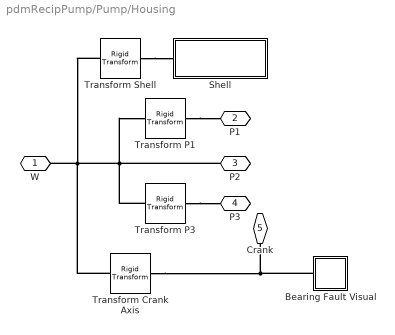
== system pdmRecipPump/Pump/Housing ==
  Bearing Fault Visual : Subsystem
  Shell : Subsystem
  Transform Crank Axis : sm_lib/Frames and Transforms/Rigid Transform  TranslationMethod=Cartesian  TranslationStandardOffset=0  TranslationLengthUnit=m  TranslationStandardAxis=+Z  TranslationCartesianOffset=crank_ax_offset  TranslationROffset=0  TranslationROffsetUnits=m  TranslationZOffset=0  TranslationZOffsetUnits=m  TranslationThetaOffset=0  TranslationThetaOffsetUnits=deg  RotationMethod=StandardAxis  RotationAngleUnits=deg  RotationStandardAxis=+Y  RotationAngle=90  RotationArbitraryAxis=[0 0 1]  FollAlignAxisA=+X  BaseAlignAxisA=+Y  FollAlignAxisB=+Y  BaseAlignAxisB=+Z  RotationSequenceAxes=FollowerAxes  RotationSequence=XYX  RotationSequenceAngles=[0 0 0]  RotationSequenceAnglesUnits=deg  RotationMatrix=[1 0 0; 0 1 0; 0 0 1]
  Transform Shell : sm_lib/Frames and Transforms/Rigid Transform  TranslationMethod=Cartesian  TranslationStandardOffset=0  TranslationLengthUnit=m  TranslationStandardAxis=+Z  TranslationCartesianOffset=TRP_Par.CAD.offset  TranslationROffset=0  TranslationROffsetUnits=m  TranslationZOffset=0  TranslationZOffsetUnits=m  TranslationThetaOffset=0  TranslationThetaOffsetUnits=deg  RotationMethod=StandardAxis  RotationAngleUnits=deg  RotationStandardAxis=+Y  RotationAngle=180  RotationArbitraryAxis=[0 0 1]  FollAlignAxisA=+X  BaseAlignAxisA=+Y  FollAlignAxisB=+Y  BaseAlignAxisB=+Z  RotationSequenceAxes=FollowerAxes  RotationSequence=XYX  RotationSequenceAngles=[0 0 0]  RotationSequenceAnglesUnits=deg  RotationMatrix=[1 0 0; 0 1 0; 0 0 1]
  Transform P1 : sm_lib/Frames and Transforms/Rigid Transform  TranslationMethod=StandardAxis  TranslationStandardOffset=-TRP_Par.Crank.Shaft.len  TranslationLengthUnit=m  TranslationStandardAxis=+X  TranslationCartesianOffset=[0 0 0]  TranslationROffset=0  TranslationROffsetUnits=m  TranslationZOffset=0  TranslationZOffsetUnits=m  TranslationThetaOffset=0  TranslationThetaOffsetUnits=deg  RotationMethod=None  RotationAngleUnits=deg  RotationStandardAxis=+Z  RotationAngle=0.0  RotationArbitraryAxis=[0 0 1]  FollAlignAxisA=+X  BaseAlignAxisA=+Y  FollAlignAxisB=+Y  BaseAlignAxisB=+Z  RotationSequenceAxes=FollowerAxes  RotationSequence=XYX  RotationSequenceAngles=[0 0 0]  RotationSequenceAnglesUnits=deg  RotationMatrix=[1 0 0; 0 1 0; 0 0 1]
  Transform P3 : sm_lib/Frames and Transforms/Rigid Transform  TranslationMethod=StandardAxis  TranslationStandardOffset=-TRP_Par.Crank.Shaft.len  TranslationLengthUnit=m  TranslationStandardAxis=-X  TranslationCartesianOffset=[0 0 0]  TranslationROffset=0  TranslationROffsetUnits=m  TranslationZOffset=0  TranslationZOffsetUnits=m  TranslationThetaOffset=0  TranslationThetaOffsetUnits=deg  RotationMethod=None  RotationAngleUnits=deg  RotationStandardAxis=+Z  RotationAngle=0.0  RotationArbitraryAxis=[0 0 1]  FollAlignAxisA=+X  BaseAlignAxisA=+Y  FollAlignAxisB=+Y  BaseAlignAxisB=+Z  RotationSequenceAxes=FollowerAxes  RotationSequence=XYX  RotationSequenceAngles=[0 0 0]  RotationSequenceAnglesUnits=deg  RotationMatrix=[1 0 0; 0 1 0; 0 0 1]
  W : PMIOPort  Side=Left
  P1 : PMIOPort  Port=2  Side=Right
  P2 : PMIOPort  Port=3  Side=Right
  P3 : PMIOPort  Port=4  Side=Right
  Crank : PMIOPort  Port=5  Side=Right
  connections:
  Transform P3/RConn1 -- P3/RConn1
  Transform P1/RConn1 -- P1/RConn1
  Transform P3/LConn1 -- Transform Shell/LConn1 -- Transform Crank Axis/LConn1 -- W/RConn1 -- P2/RConn1 -- Transform P1/LConn1
  Transform Shell/RConn1 -- Shell/LConn1
  Transform Crank Axis/RConn1 -- Bearing Fault Visual/LConn1 -- Crank/RConn1
